simulink model "simulink_model"  (R2025b)
settings: Solver=VariableStepAuto  StartTime=0.0  StopTime=20  RelTol=1e-3
settings Model: Creator=leonard  LastModifiedBy=leonard

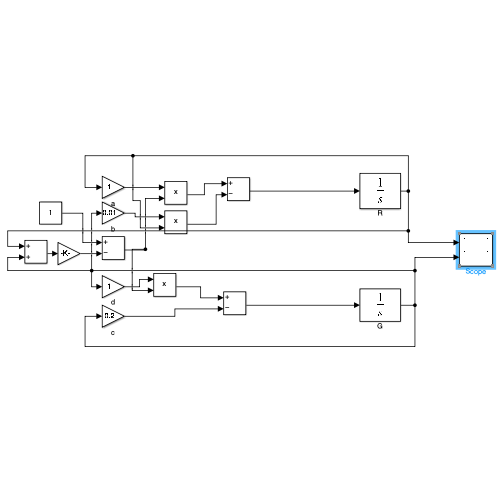
[thumbnail: Simulink's stored preview of the top-level diagram]
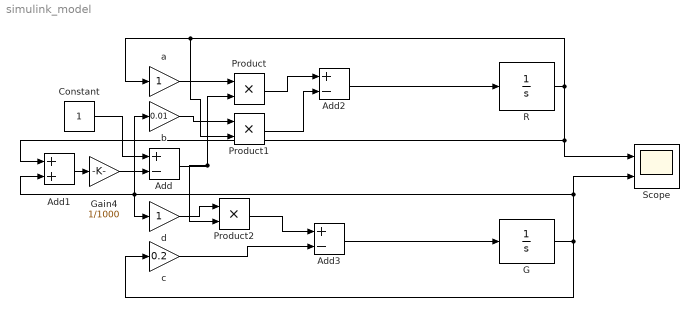
== system simulink_model ==
  Add : Sum  Inputs=+-
  Add1 : Sum
  Add2 : Sum  Inputs=+-
  Add3 : Sum  Inputs=+-
  Constant : Constant
  G : Integrator  InitialCondition=10
  Gain4 : Gain  Gain=1/1000
  Product : Product
  Product1 : Product
  Product2 : Product
  R : Integrator  InitialCondition=200
  Scope : Scope  NumInputPorts=2
      settings: ActiveDisplayYMinimum=-99.866438134067181  ActiveDisplayYMaximum=898.797943797362
  a : Gain
  b : Gain  Gain=0.01
  c : Gain  Gain=0.2
  d : Gain
  wires:
  Constant/1 -> Add/1
  Add1/1 -> Gain4/1
  Gain4/1 -> Add/2
  Add2/1 -> R/1
  Add3/1 -> G/1
  R/1 -> Scope/1, Add1/1, Product1/2, a/1
  a/1 -> Product/1
  G/1 -> Scope/2, d/1, b/1, Add1/2, c/1
  Add/1 -> Product2/2, Product/2
  Product/1 -> Add2/1
  b/1 -> Product1/1
  Product1/1 -> Add2/2
  c/1 -> Add3/2
  Product2/1 -> Add3/1
  d/1 -> Product2/1
